simulink model "InvertedPendulum"  (R2024b)
settings: Solver=VariableStepAuto  StartTime=0.0  StopTime=10.0  RelTol=1e-3
model workspace (MAT data in the model file):
  Sig = Simulink.Signal
  Sig.Dimensions = -1
  Sig.DimensionsMode = 'auto'
  Sig.Complexity = 'auto'
  Sig.SampleTime = -1
  Sig.SamplingMode = 'auto'
  Sig.DataType = 'auto'
settings Model: Creator=nopla  LastModifiedBy=nopla

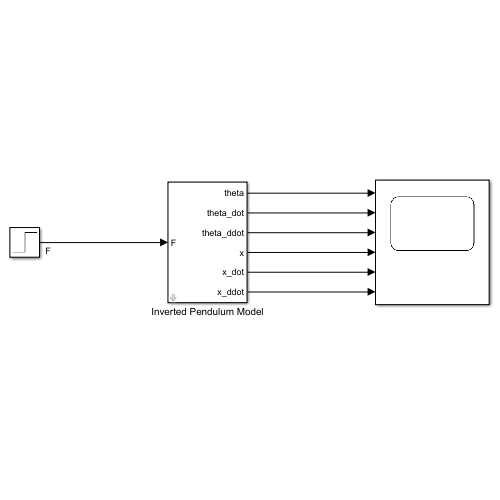
[thumbnail: Simulink's stored preview of the top-level diagram]
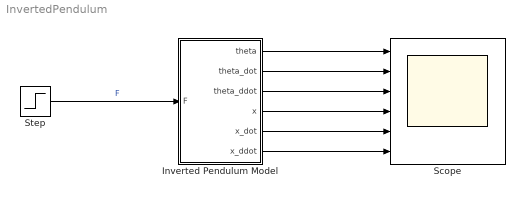
== system InvertedPendulum ==
  Inverted Pendulum Model : Subsystem  mask{CartMass=0.5, PendulumMass=0.2, PendulumLength=0.3, PendulumInertia=0.05, g=9.81}
      mask DialogControl ParameterGroupVar Prompt: パラメーター
  Scope : Scope  NumInputPorts=6
  Step : Step  SampleTime=0
  wires:
  Step/1 -> Inverted Pendulum Model/1(F)  "F"
  Inverted Pendulum Model/1(theta) -> Scope/1
  Inverted Pendulum Model/2(theta_dot) -> Scope/2
  Inverted Pendulum Model/3(theta_ddot) -> Scope/3
  Inverted Pendulum Model/4(x) -> Scope/4
  Inverted Pendulum Model/5(x_dot) -> Scope/5
  Inverted Pendulum Model/6(x_ddot) -> Scope/6

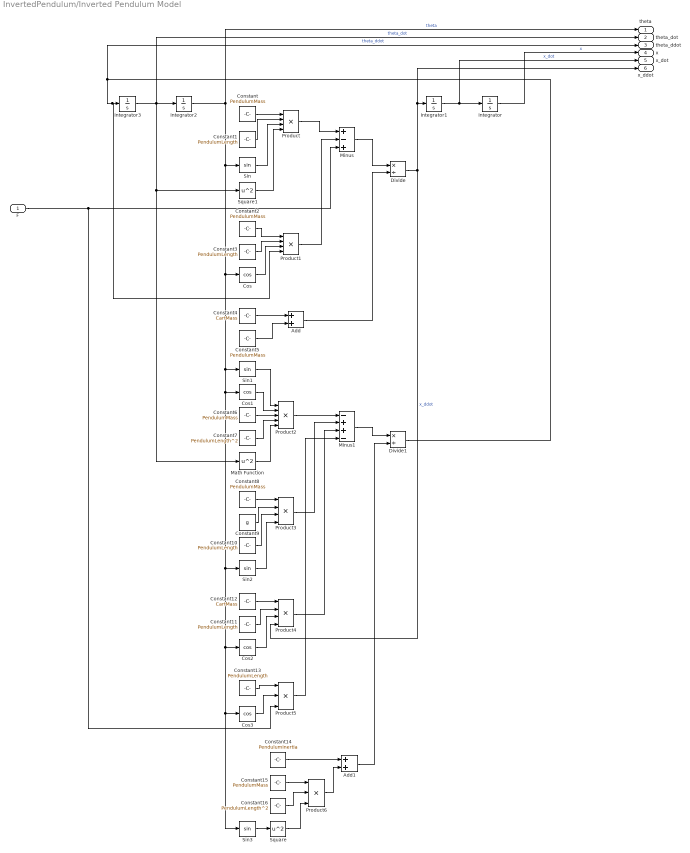
== system InvertedPendulum/Inverted Pendulum Model ==
  F : Inport
  Add : Sum
  Add1 : Sum
  Constant{,2,5..6,8,15} (6 alike) : Constant  Value=PendulumMass
  Constant{1,3,10..11,13} (5 alike) : Constant  Value=PendulumLength
  Constant12 : Constant  Value=CartMass
  Constant14 : Constant  Value=PendulumInertia
  Constant16 : Constant  Value=PendulumLength^2
  Constant4 : Constant  Value=CartMass
  Constant7 : Constant  Value=PendulumLength^2
  Constant9 : Constant  Value=g
  Cos{,1..3} (4 alike) : Trigonometry  Operator=cos
  Divide : Product  Inputs=*/
  Divide1 : Product  Inputs=*/
  Integrator{,1..3} (4 alike) : Integrator
  Math Function : Math  Operator=square
  Minus : Sum  Inputs=+-+
  Minus1 : Sum  Inputs=-++-
  Product{,1,3..4} (4 alike) : Product  Inputs=4
  Product2 : Product  Inputs=5
  Product5 : Product  Inputs=3
  Product6 : Product  Inputs=3
  Sin{,1..3} (4 alike) : Trigonometry
  Square : Math  Operator=square
  Square1 : Math  Operator=square
  theta : Outport
  theta_dot : Outport  Port=2
  theta_ddot : Outport  Port=3
  x : Outport  Port=4
  x_dot : Outport  Port=5
  x_ddot : Outport  Port=6
  wires:
  Square/1 -> Product6/3
  Integrator2/1 -> theta/1, Cos2/1, Sin3/1, Cos3/1, Sin2/1, Cos1/1, Sin1/1, Cos/1, Sin/1  "theta"
  Product6/1 -> Add1/2
  Sin2/1 -> Product3/4
  Minus1/1 -> Divide1/1
  Integrator3/1 -> theta_dot/1, Math Function/1, Square1/1, Integrator2/1  "theta_dot"
  Constant15/1 -> Product6/1
  Cos/1 -> Product1/3
  Constant10/1 -> Product3/3
  Cos2/1 -> Product4/3
  Constant12/1 -> Product4/1
  Constant1/1 -> Product/2
  Divide/1 -> Product4/4, x_ddot/1, Integrator1/1  "x_ddot"
  F/1 -> Minus/3, Product5/3
  Integrator/1 -> x/1  "x"
  Constant3/1 -> Product1/2
  Integrator1/1 -> x_dot/1, Integrator/1  "x_dot"
  Sin3/1 -> Square/1
  Product2/1 -> Minus1/1
  Product5/1 -> Minus1/4
  Constant16/1 -> Product6/2
  Constant4/1 -> Add/1
  Product1/1 -> Minus/2
  Constant7/1 -> Product2/4
  Constant9/1 -> Product3/2
  Product3/1 -> Minus1/2
  Add1/1 -> Divide1/2
  Square1/1 -> Product/4
  Sin1/1 -> Product2/1
  Constant/1 -> Product/1
  Sin/1 -> Product/3
  Cos3/1 -> Product5/2
  Divide1/1 -> theta_ddot/1, Integrator3/1, Product1/4  "theta_ddot"
  Constant5/1 -> Add/2
  Constant14/1 -> Add1/1
  Add/1 -> Divide/2
  Constant2/1 -> Product1/1
  Math Function/1 -> Product2/5
  Product/1 -> Minus/1
  Constant8/1 -> Product3/1
  Minus/1 -> Divide/1
  Constant11/1 -> Product4/2
  Constant6/1 -> Product2/3
  Product4/1 -> Minus1/3
  Cos1/1 -> Product2/2
  Constant13/1 -> Product5/1
